simulink model "Projekt"  (R2013a)
settings: Solver=ode45  StartTime=0.0  StopTime=10  RelTol=1e-3
values from neighbouring files (symbols this model uses):
  P_0 = reshape(P_0,9,1)    [init.m]
  q0_est = [cos(pi/3);sin(pi/3)/(3)^0.5;-sin(pi/3)/(3)^0.5;sin(pi/3)/(3)^0.5]    [init.m]
  q1 = multiply(q_inv,q_y)-[1;0;0;0]    [Kalman.m]    (also in init.m = [1; 0; 0; 0]; obiekt.m = vals(5:8))
libraries: simulink x3
settings Model: Creator=Ula  LastModifiedBy=Ula
settings DataIOCC: SignalLoggingSaveFormat=ModelDataLogs
settings OptimizationCC: InitFltsAndDblsToZero=on
settings DebuggingCC: SaveWithParameterizedLinksMsg=none  SignalResolutionControl=TryResolveAllWithWarning  MultiTaskDSMMsg=warning  MultiTaskCondExecSysMsg=none  FcnCallInpInsideContextMsg=UseLocalSettings  StrictBusMsg=Warning
settings RTWCC: IncludeERTFirstTime=on
settings GRTTargetCC: TargetFcnLib=ansi_tfl_tmw.mat  CombineOutputUpdateFcns=off  GRTInterface=on

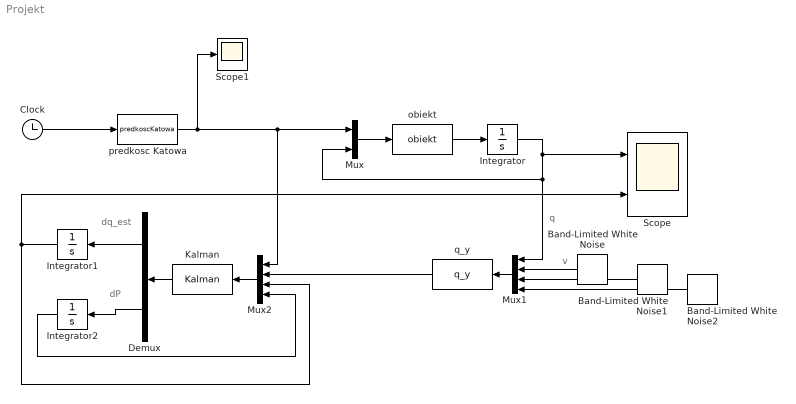
== system Projekt ==
  note: q
  note: v
  note: dq_est
  note: dP
  Band-Limited White Noise : simulink/Sources/Band-Limited White Noise  Cov=[0.1]  Ts=0.1  seed=[21941]
  Band-Limited White Noise1 : simulink/Sources/Band-Limited White Noise  Cov=[0.1]  Ts=0.1  seed=[25671]
  Band-Limited White Noise2 : simulink/Sources/Band-Limited White Noise  Cov=[0.1]  Ts=0.1  seed=[18341]
  Clock : Clock
  Demux : Demux  Outputs=[4 9]
  Integrator : Integrator  InitialCondition=q1
  Integrator1 : Integrator  InitialCondition=q0_est
  Integrator2 : Integrator  InitialCondition=P_0
  Kalman : MATLABFcn  MATLABFcn=Kalman
  Mux : Mux  Inputs=2
  Mux1 : Mux
  Mux2 : Mux
  Scope : Scope  NumInputPorts=2
      settings: YMin=-5~-5  YMax=5~5
  Scope1 : Scope
  obiekt : MATLABFcn  MATLABFcn=obiekt
  predkosc Katowa : MATLABFcn  MATLABFcn=predkoscKatowa
  q_y : MATLABFcn  MATLABFcn=q_y
  wires:
  Mux/1 -> obiekt/1
  Clock/1 -> predkosc Katowa/1
  predkosc Katowa/1 -> Scope1/1, Mux/1, Mux2/1
  obiekt/1 -> Integrator/1
  Integrator/1 -> Mux1/1, Mux/2, Scope/1
  Band-Limited White Noise/1 -> Mux1/2
  Band-Limited White Noise1/1 -> Mux1/3
  Band-Limited White Noise2/1 -> Mux1/4
  Mux1/1 -> q_y/1
  q_y/1 -> Mux2/2
  Mux2/1 -> Kalman/1
  Kalman/1 -> Demux/1
  Demux/1 -> Integrator1/1
  Demux/2 -> Integrator2/1
  Integrator1/1 -> Scope/2, Mux2/3
  Integrator2/1 -> Mux2/4
